simulink model "F16_aero"  (Simulink 7.2)
settings: Solver=ode45  StartTime=0.0  StopTime=10.0  RelTol=1e-3
model workspace (MAT data in the model file):
  F16_aero_data.ALPHA1_pts = [-10 -5 0 5 10 15 20 25 30 35 40 45]
  F16_aero_data.CX_table = [-0.099  -0.081  -0.081  -0.063  -0.025  0.044  0.097  0.113  0.145  0.167  0.174  0.166; -0.048  -0.038  -0.04  -0.021  0.016  0.083  0.127  0.137  0.162  0.177  0.179  0.167; -0.022  -0.02  -0.021  -0.004  0.032  0.094  0.128  0.13  0.154  0.161  0.155  0.138; -0.04  -0.038  -0.039  -0.025  0.006  0.062  0.087  0.085  0.1  0.11  0.104  0.091; -0.083  -0.073  -0.076  -0.072  -0.046  0.012  0.024  0.025  0.043  0.053  0.047  0.04]
  F16_aero_data.CZ0_table = [0.77 0.241 -0.1 -0.416 -0.731 -1.053 -1.366 -1.646 -1.917 -2.12 -2.248 -2.229]
  F16_aero_data.Cm0_table = [0.205  0.168  0.186  0.196  0.213  0.251  0.245  0.238  0.252  0.231  0.198  0.192; 0.081  0.077  0.107  0.11  0.11  0.141  0.127  0.119  0.133  0.108  0.081  0.093; -0.046  -0.02  -0.009  -0.005  -0.006  0.01  0.006  -0.001  0.014  0  -0.013  0.032; -0.174  -0.145  -0.121  -0.127  -0.129  -0.102  -0.097  -0.113  -0.087  -0.084  -0.069  -0.006; -0.259  -0.202  -0.184  -0.193  -0.199  -0.15  -0.16  -0.167  -0.104  -0.076  -0.041  -0.005]
  F16_aero_data.Cl0_table = [0  0  0  0  0  0  0  0  0  0  0  0; -0.001  -0.004  -0.008  -0.012  -0.016  -0.022  -0.022  -0.021  -0.015  -0.008  -0.013  -0.015; -0.003  -0.009  -0.017  -0.024  -0.03  -0.041  -0.045  -0.04  -0.016  -0.002  -0.01  -0.019; -0.001  -0.01  -0.02  -0.03  -0.039  -0.054  -0.057  -0.054  -0.023  -0.006  -0.014  -0.027; 0  -0.01  -0.022  -0.034  -0.047  -0.06  -0.069  -0.067  -0.033  -0.036  -0.035  -0.035; 0.007  -0.01  -0.023  -0.034  -0.049  -0.063  -0.081  -0.079  -0.06  -0.058  -0.062  -0.059; 0.009  -0.011  -0.023  -0.037  -0.05  -0.068  -0.089  -0.088  -0.091  -0.076  -0.077  -0.076]
  F16_aero_data.Cn0_table = [0  0  0  0  0  0  0  0  0  0  0  0; 0.018  0.019  0.018  0.019  0.019  0.018  0.013  0.007  0.004  -0.014  -0.017  -0.033; 0.038  0.042  0.042  0.042  0.043  0.039  0.03  0.017  0.004  -0.035  -0.047  -0.057; 0.056  0.057  0.059  0.058  0.058  0.053  0.032  0.012  0.002  -0.046  -0.071  -0.073; 0.064  0.077  0.076  0.074  0.073  0.057  0.029  0.007  0.012  -0.034  -0.065  -0.041; 0.074  0.086  0.093  0.089  0.08  0.062  0.049  0.022  0.028  -0.012  -0.002  -0.013; 0.079  0.09  0.106  0.106  0.096  0.08  0.068  0.03  0.064  0.015  0.011  -0.001]
  F16_aero_data.CXq_table = [-0.267 -0.11 0.308 1.34 2.08 2.91 2.76 2.05 1.5 1.49 1.83 1.21]
  F16_aero_data.CYr_table = [0.882 0.852 0.876 0.958 0.962 0.974 0.819 0.483 0.59 1.21 -0.493 -1.04]
  F16_aero_data.CYp_table = [-0.108 -0.108 -0.188 0.11 0.258 0.226 0.344 0.362 0.611 0.529 0.298 -0.227]
  F16_aero_data.CZq_table = [-8.8 -25.8 -28.9 -31.4 -31.2 -30.7 -27.7 -28.2 -29 -29.8 -38.3 -35.3]
  F16_aero_data.Clr_table = [-0.126 -0.026 0.063 0.113 0.208 0.23 0.319 0.437 0.68 0.1 0.447 -0.33]
  F16_aero_data.Clp_table = [-0.36 -0.359 -0.443 -0.42 -0.383 -0.375 -0.329 -0.294 -0.23 -0.21 -0.12 -0.1]
  F16_aero_data.Cmq_table = [-7.21 -5.4 -5.23 -5.26 -6.11 -6.64 -5.69 -6 -6.2 -6.4 -6.6 -6]
  F16_aero_data.Cnr_table = [-0.38 -0.363 -0.378 -0.386 -0.37 -0.453 -0.55 -0.582 -0.595 -0.637 -1.02 -0.84]
  F16_aero_data.Cnp_table = [0.061 0.052 0.052 -0.012 -0.013 -0.024 0.05 0.15 0.13 0.158 0.24 0.15]
  F16_aero_data.dlda_table = [-0.041  -0.052  -0.053  -0.056  -0.05  -0.056  -0.082  -0.059  -0.042  -0.038  -0.027  -0.017; -0.041  -0.053  -0.053  -0.053  -0.05  -0.051  -0.066  -0.043  -0.038  -0.027  -0.023  -0.016; -0.042  -0.053  -0.052  -0.051  -0.049  -0.049  -0.043  -0.035  -0.026  -0.016  -0.018  -0.014; -0.04  -0.052  -0.051  -0.052  -0.048  -0.048  -0.042  -0.037  -0.031  -0.026  -0.017  -0.012; -0.043  -0.049  -0.048  -0.049  -0.043  -0.042  -0.042  -0.036  -0.025  -0.021  -0.016  -0.011; -0.044  -0.048  -0.048  -0.047  -0.042  -0.041  -0.02  -0.028  -0.013  -0.014  -0.011  -0.01; -0.043  -0.049  -0.047  -0.045  -0.042  -0.037  -0.003  -0.013  -0.01  -0.003  -0.007  -0.008]
  F16_aero_data.dldr_table = [0.005  0.017  0.014  0.01  -0.005  0.009  0.019  0.005  0  -0.005  -0.011  0.008; 0.007  0.016  0.014  0.014  0.013  0.009  0.012  0.005  0  0.004  0.009  0.007; 0.013  0.013  0.011  0.012  0.011  0.009  0.008  0.005  0  0.005  0.003  0.005; 0.018  0.015  0.015  0.014  0.014  0.014  0.014  0.015  0.013  0.011  0.006  0.001; 0.015  0.014  0.013  0.013  0.012  0.011  0.011  0.01  0.008  0.008  0.007  0.003; 0.021  0.011  0.01  0.011  0.01  0.009  0.008  0.01  0.006  0.005  0  0.001; 0.023  0.01  0.011  0.011  0.011  0.01  0.008  0.01  0.006  0.014  0.02  0]
  F16_aero_data.dnda_table = [0.001  -0.027  -0.017  -0.013  -0.012  -0.016  0.001  0.017  0.011  0.017  0.008  0.016; 0.002  -0.014  -0.016  -0.016  -0.014  -0.019  -0.021  0.002  0.012  0.016  0.015  0.011; -0.006  -0.008  -0.006  -0.006  -0.005  -0.008  -0.005  0.007  0.004  0.007  0.006  0.006; -0.011  -0.011  -0.01  -0.009  -0.008  -0.006  0  0.004  0.007  0.01  0.004  0.01; -0.015  -0.015  -0.014  -0.012  -0.011  -0.008  -0.002  0.002  0.006  0.012  0.011  0.011; -0.024  -0.01  -0.004  -0.002  -0.001  0.003  0.014  0.006  -0.001  0.004  0.004  0.006; -0.022  0.002  -0.003  -0.005  -0.003  -0.001  -0.009  -0.009  -0.001  0.003  -0.002  0.001]
  F16_aero_data.dndr_table = [-0.018  -0.052  -0.052  -0.052  -0.054  -0.049  -0.059  -0.051  -0.03  -0.037  -0.026  -0.013; -0.028  -0.051  -0.043  -0.046  -0.045  -0.049  -0.057  -0.052  -0.03  -0.033  -0.03  -0.008; -0.037  -0.041  -0.038  -0.04  -0.04  -0.038  -0.037  -0.03  -0.027  -0.024  -0.019  -0.013; -0.048  -0.045  -0.045  -0.045  -0.044  -0.045  -0.047  -0.048  -0.049  -0.045  -0.033  -0.016; -0.043  -0.044  -0.041  -0.041  -0.04  -0.038  -0.034  -0.035  -0.035  -0.029  -0.022  -0.009; -0.052  -0.034  -0.036  -0.036  -0.035  -0.028  -0.024  -0.023  -0.02  -0.016  -0.01  -0.014; -0.062  -0.034  -0.027  -0.028  -0.027  -0.027  -0.023  -0.023  -0.019  -0.009  -0.025  -0.01]
  F16_aero_data.BETA2_pts = [-30 -20 -10 0 10 20 30]
  F16_aero_data.BETA1_pts = [0 5 10 15 20 25 30]
  F16_aero_data.DE1_pts : numeric (value not decoded)
libraries: simulink_need_slupdate x22
settings Model: Creator=bjax  LastModifiedBy=bjax

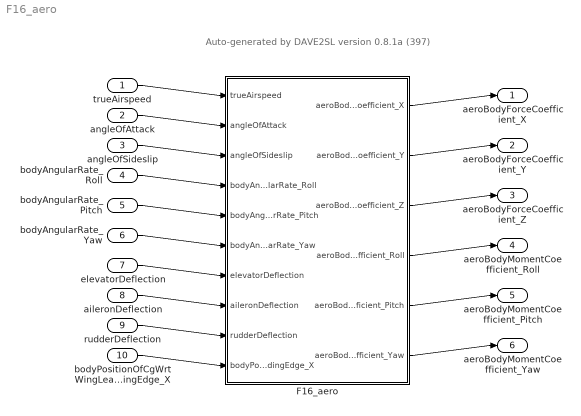
== system F16_aero ==
  note: Auto-generated by DAVE2SL version 0.8.1a (397)
  trueAirspeed : Inport
  angleOfAttack : Inport  Port=2
  angleOfSideslip : Inport  Port=3
  bodyAngularRate_Roll : Inport  Port=4
  bodyAngularRate_Pitch : Inport  Port=5
  bodyAngularRate_Yaw : Inport  Port=6
  elevatorDeflection : Inport  Port=7
  aileronDeflection : Inport  Port=8
  rudderDeflection : Inport  Port=9
  bodyPositionOfCgWrtWingLeadingEdge_X : Inport  Port=10
  F16_aero : Subsystem
  aeroBodyForceCoefficient_X : Outport
  aeroBodyForceCoefficient_Y : Outport  Port=2
  aeroBodyForceCoefficient_Z : Outport  Port=3
  aeroBodyMomentCoefficient_Roll : Outport  Port=4
  aeroBodyMomentCoefficient_Pitch : Outport  Port=5
  aeroBodyMomentCoefficient_Yaw : Outport  Port=6
  wires:
  trueAirspeed/1 -> F16_aero/1(trueAirspeed)
  angleOfAttack/1 -> F16_aero/2(angleOfAttack)
  angleOfSideslip/1 -> F16_aero/3(angleOfSideslip)
  bodyAngularRate_Roll/1 -> F16_aero/4(bodyAngularRate_Roll)
  bodyAngularRate_Pitch/1 -> F16_aero/5(bodyAngularRate_Pitch)
  bodyAngularRate_Yaw/1 -> F16_aero/6(bodyAngularRate_Yaw)
  elevatorDeflection/1 -> F16_aero/7(elevatorDeflection)
  aileronDeflection/1 -> F16_aero/8(aileronDeflection)
  rudderDeflection/1 -> F16_aero/9(rudderDeflection)
  bodyPositionOfCgWrtWingLeadingEdge_X/1 -> F16_aero/10(bodyPositionOfCgWrtWingLeadingEdge_X)
  F16_aero/1(aeroBodyForceCoefficient_X) -> aeroBodyForceCoefficient_X/1
  F16_aero/2(aeroBodyForceCoefficient_Y) -> aeroBodyForceCoefficient_Y/1
  F16_aero/3(aeroBodyForceCoefficient_Z) -> aeroBodyForceCoefficient_Z/1
  F16_aero/4(aeroBodyMomentCoefficient_Roll) -> aeroBodyMomentCoefficient_Roll/1
  F16_aero/5(aeroBodyMomentCoefficient_Pitch) -> aeroBodyMomentCoefficient_Pitch/1
  F16_aero/6(aeroBodyMomentCoefficient_Yaw) -> aeroBodyMomentCoefficient_Yaw/1

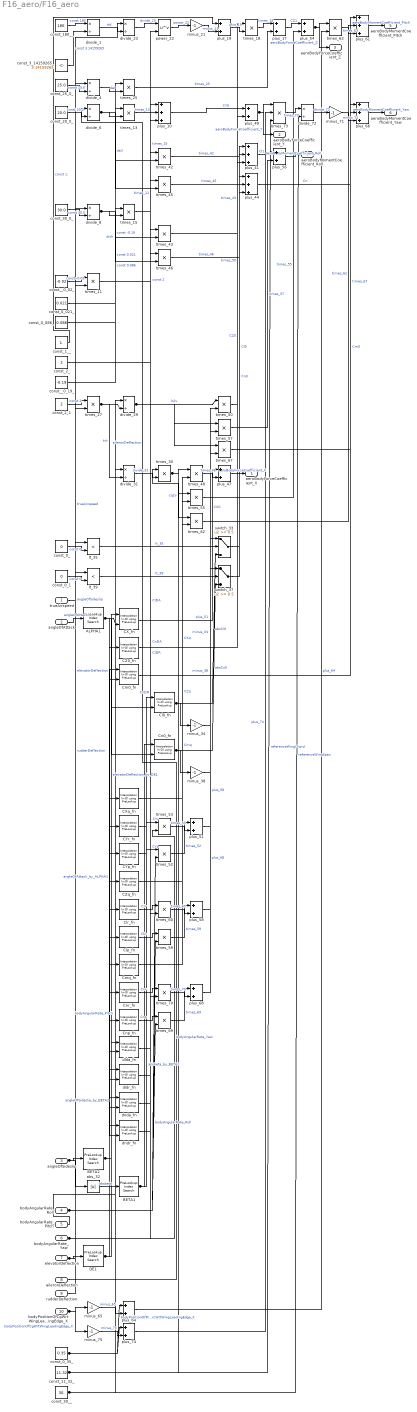
== system F16_aero/F16_aero ==
  trueAirspeed : Inport
  angleOfAttack : Inport  Port=2
  angleOfSideslip : Inport  Port=3
  bodyAngularRate_Roll : Inport  Port=4
  bodyAngularRate_Pitch : Inport  Port=5
  bodyAngularRate_Yaw : Inport  Port=6
  elevatorDeflection : Inport  Port=7
  aileronDeflection : Inport  Port=8
  rudderDeflection : Inport  Port=9
  bodyPositionOfCgWrtWingLeadingEdge_X : Inport  Port=10
  ALPHA1 : simulink_need_slupdate/PreLookup Index Search  bpData=F16_aero_data.ALPHA1_pts  searchMode=Binary Search  cacheBpFlag=on  outputFlag=off  IndexDataType=uint32  extrapMode=Linear Extrapolation  rangeErrorMode=None
  BETA1 : simulink_need_slupdate/PreLookup Index Search  bpData=F16_aero_data.BETA1_pts  searchMode=Binary Search  cacheBpFlag=on  outputFlag=off  IndexDataType=uint32  extrapMode=Linear Extrapolation  rangeErrorMode=None
  BETA2 : simulink_need_slupdate/PreLookup Index Search  bpData=F16_aero_data.BETA2_pts  searchMode=Binary Search  cacheBpFlag=on  outputFlag=off  IndexDataType=uint32  extrapMode=Linear Extrapolation  rangeErrorMode=None
  CX_fn : simulink_need_slupdate/Interpolation (n-D) using PreLookup  numDimsPopupSelect=2  explicitNumDims=2  table=F16_aero_data.CX_table  interpMethod=Linear  extrapMethod=None - Clip  rangeErrorMode=None  NumSelectionDims=0
  CXq_fn : simulink_need_slupdate/Interpolation (n-D) using PreLookup  numDimsPopupSelect=1  explicitNumDims=1  table=F16_aero_data.CXq_table  interpMethod=Linear  extrapMethod=None - Clip  rangeErrorMode=None  NumSelectionDims=0
  CYp_fn : simulink_need_slupdate/Interpolation (n-D) using PreLookup  numDimsPopupSelect=1  explicitNumDims=1  table=F16_aero_data.CYp_table  interpMethod=Linear  extrapMethod=None - Clip  rangeErrorMode=None  NumSelectionDims=0
  CYr_fn : simulink_need_slupdate/Interpolation (n-D) using PreLookup  numDimsPopupSelect=1  explicitNumDims=1  table=F16_aero_data.CYr_table  interpMethod=Linear  extrapMethod=None - Clip  rangeErrorMode=None  NumSelectionDims=0
  CZ0_fn : simulink_need_slupdate/Interpolation (n-D) using PreLookup  numDimsPopupSelect=1  explicitNumDims=1  table=F16_aero_data.CZ0_table  interpMethod=Linear  extrapMethod=None - Clip  rangeErrorMode=None  NumSelectionDims=0
  CZq_fn : simulink_need_slupdate/Interpolation (n-D) using PreLookup  numDimsPopupSelect=1  explicitNumDims=1  table=F16_aero_data.CZq_table  interpMethod=Linear  extrapMethod=None - Clip  rangeErrorMode=None  NumSelectionDims=0
  Cl0_fn : simulink_need_slupdate/Interpolation (n-D) using PreLookup  numDimsPopupSelect=2  explicitNumDims=2  table=F16_aero_data.Cl0_table  interpMethod=Linear  extrapMethod=None - Clip  rangeErrorMode=None  NumSelectionDims=0
  Clp_fn : simulink_need_slupdate/Interpolation (n-D) using PreLookup  numDimsPopupSelect=1  explicitNumDims=1  table=F16_aero_data.Clp_table  interpMethod=Linear  extrapMethod=None - Clip  rangeErrorMode=None  NumSelectionDims=0
  Clr_fn : simulink_need_slupdate/Interpolation (n-D) using PreLookup  numDimsPopupSelect=1  explicitNumDims=1  table=F16_aero_data.Clr_table  interpMethod=Linear  extrapMethod=None - Clip  rangeErrorMode=None  NumSelectionDims=0
  Cm0_fn : simulink_need_slupdate/Interpolation (n-D) using PreLookup  numDimsPopupSelect=2  explicitNumDims=2  table=F16_aero_data.Cm0_table  interpMethod=Linear  extrapMethod=None - Clip  rangeErrorMode=None  NumSelectionDims=0
  Cmq_fn : simulink_need_slupdate/Interpolation (n-D) using PreLookup  numDimsPopupSelect=1  explicitNumDims=1  table=F16_aero_data.Cmq_table  interpMethod=Linear  extrapMethod=None - Clip  rangeErrorMode=None  NumSelectionDims=0
  Cn0_fn : simulink_need_slupdate/Interpolation (n-D) using PreLookup  numDimsPopupSelect=2  explicitNumDims=2  table=F16_aero_data.Cn0_table  interpMethod=Linear  extrapMethod=None - Clip  rangeErrorMode=None  NumSelectionDims=0
  Cnp_fn : simulink_need_slupdate/Interpolation (n-D) using PreLookup  numDimsPopupSelect=1  explicitNumDims=1  table=F16_aero_data.Cnp_table  interpMethod=Linear  extrapMethod=None - Clip  rangeErrorMode=None  NumSelectionDims=0
  Cnr_fn : simulink_need_slupdate/Interpolation (n-D) using PreLookup  numDimsPopupSelect=1  explicitNumDims=1  table=F16_aero_data.Cnr_table  interpMethod=Linear  extrapMethod=None - Clip  rangeErrorMode=None  NumSelectionDims=0
  DE1 : simulink_need_slupdate/PreLookup Index Search  bpData=F16_aero_data.DE1_pts  searchMode=Binary Search  cacheBpFlag=on  outputFlag=off  IndexDataType=uint32  extrapMode=Linear Extrapolation  rangeErrorMode=None
  abs_32 : Abs  SaturateOnIntegerOverflow=on
  const_0_ : Constant  Value=0
  const_0_021_ : Constant  Value=0.021
  const_0_086_ : Constant  Value=0.086
  const_0_1 : Constant  Value=0
  const_0_35_ : Constant  Value=0.35
  const_11_32_ : Constant  Value=11.32
  const_180__ : Constant  Value=180.
  const_1__ : Constant  Value=1.
  const_20_0_ : Constant  Value=20.0
  const_25_0_ : Constant  Value=25.0
  const_2_ : Constant  Value=2
  const_2_1 : Constant  Value=2
  const_30_0_ : Constant  Value=30.0
  const_30__ : Constant  Value=30.
  const_3_14159265_ : Constant  Value=3.14159265
  const__0_02_ : Constant  Value=-0.02
  const__0_19_ : Constant  Value=-0.19
  divide_{1,4,6,8,23,29,31,72} (8 alike) : Product  Inputs=*/  SaturateOnIntegerOverflow=on  RndMeth=Zero  InputSameDT=on  OutDataTypeStr=Inherit: Same as first input
  dlda_fn : simulink_need_slupdate/Interpolation (n-D) using PreLookup  numDimsPopupSelect=2  explicitNumDims=2  table=F16_aero_data.dlda_table  interpMethod=Linear  extrapMethod=None - Clip  rangeErrorMode=None  NumSelectionDims=0
  dldr_fn : simulink_need_slupdate/Interpolation (n-D) using PreLookup  numDimsPopupSelect=2  explicitNumDims=2  table=F16_aero_data.dldr_table  interpMethod=Linear  extrapMethod=None - Clip  rangeErrorMode=None  NumSelectionDims=0
  dnda_fn : simulink_need_slupdate/Interpolation (n-D) using PreLookup  numDimsPopupSelect=2  explicitNumDims=2  table=F16_aero_data.dnda_table  interpMethod=Linear  extrapMethod=None - Clip  rangeErrorMode=None  NumSelectionDims=0
  dndr_fn : simulink_need_slupdate/Interpolation (n-D) using PreLookup  numDimsPopupSelect=2  explicitNumDims=2  table=F16_aero_data.dndr_table  interpMethod=Linear  extrapMethod=None - Clip  rangeErrorMode=None  NumSelectionDims=0
  lt_35 : RelationalOperator  Operator=<  InputSameDT=on
  lt_39 : RelationalOperator  Operator=<  InputSameDT=on
  minus_{21,34,38,65,71,75} (6 alike) : Gain  Gain=-1  SaturateOnIntegerOverflow=on  OutDataTypeStr=Inherit: Same as input  ParamDataTypeStr=Inherit: Same as input
  plus_{10,41,44,61,66} (5 alike) : Sum  Inputs=+++  SaturateOnIntegerOverflow=on  InputSameDT=on  OutDataTypeStr=Inherit: Same as first input
  plus_{17,19,47,49,51,54,56,58,64,68,74} (11 alike) : Sum  SaturateOnIntegerOverflow=on  InputSameDT=on  OutDataTypeStr=Inherit: Same as first input
  power_22 : Math  Operator=pow  SaturateOnIntegerOverflow=on
  switch_33 : Switch  Threshold=0.5  SaturateOnIntegerOverflow=on  InputSameDT=on
  switch_37 : Switch  Threshold=0.5  SaturateOnIntegerOverflow=on  InputSameDT=on
  times_{11,13,15,18,25,27,30,42..43,45..46,48,50,52..53,55,57,59..60,62..63,67,69..70} (24 alike) : Product  SaturateOnIntegerOverflow=on  RndMeth=Zero  InputSameDT=on  OutDataTypeStr=Inherit: Same as first input
  times_73 : Product  Inputs=3  SaturateOnIntegerOverflow=on  RndMeth=Zero  InputSameDT=on  OutDataTypeStr=Inherit: Same as first input
  aeroBodyForceCoefficient_X : Outport
  aeroBodyForceCoefficient_Y : Outport  Port=2
  aeroBodyForceCoefficient_Z : Outport  Port=3
  aeroBodyMomentCoefficient_Roll : Outport  Port=4
  aeroBodyMomentCoefficient_Pitch : Outport  Port=5
  aeroBodyMomentCoefficient_Yaw : Outport  Port=6
  wires:
  trueAirspeed/1 -> times_27/2  "trueAirspeed"
  angleOfAttack/1 -> ALPHA1/1  "angleOfAttack"
  angleOfSideslip/1 -> BETA2/1, times_11/2, divide_23/1, abs_32/1, lt_35/1, lt_39/1  "angleOfSideslip"
  bodyAngularRate_Roll/1 -> times_52/2, times_59/2, times_69/2  "bodyAngularRate_Roll"
  bodyAngularRate_Pitch/1 -> divide_31/1  "bodyAngularRate_Pitch"
  bodyAngularRate_Yaw/1 -> times_53/2, times_60/2, times_70/2  "bodyAngularRate_Yaw"
  elevatorDeflection/1 -> DE1/1, divide_4/1  "elevatorDeflection"
  aileronDeflection/1 -> divide_6/1  "aileronDeflection"
  rudderDeflection/1 -> divide_8/1  "rudderDeflection"
  bodyPositionOfCgWrtWingLeadingEdge_X/1 -> minus_65/1, minus_75/1  "bodyPositionOfCgWrtWingLeadingEdge_X"
  divide_1/1 -> divide_23/2  "rtd"
  const_180__/1 -> divide_1/1  "const 180."
  const_3_14159265_/1 -> divide_1/2  "const 3.14159265"
  const_0_35_/1 -> plus_64/1, plus_74/1  "bodyPositionOfMrcWrtWingLeadingEdge_X"
  const_11_32_/1 -> times_30/1, times_73/3  "referenceWingChord"
  const_30__/1 -> divide_29/1, divide_72/2  "referenceWingSpan"
  divide_4/1 -> times_25/2  "del"
  const_25_0_/1 -> divide_4/2  "const 25.0"
  divide_6/1 -> times_13/2, times_42/2, times_45/2  "dail"
  const_20_0_/1 -> divide_6/2  "const 20.0"
  divide_8/1 -> times_15/2, times_43/2, times_46/2  "drdr"
  const_30_0_/1 -> divide_8/2  "const 30.0"
  CX_fn/1 -> plus_47/1  "CX0"
  plus_10/1 -> plus_49/1  "CY0"
  times_11/1 -> plus_10/1  "times_11"
  const__0_02_/1 -> times_11/1  "const -0.02"
  times_13/1 -> plus_10/2  "times_13"
  const_0_021_/1 -> times_13/1  "const 0.021"
  times_15/1 -> plus_10/3  "times_15"
  const_0_086_/1 -> times_15/1  "const 0.086"
  CZ0_fn/1 -> times_18/1  "CZ0"
  plus_17/1 -> plus_54/1  "CZ1"
  times_18/1 -> plus_17/1  "times_18"
  plus_19/1 -> times_18/2  "plus_19"
  const_1__/1 -> plus_19/1  "const 1."
  minus_21/1 -> plus_19/2  "minus_21"
  power_22/1 -> minus_21/1  "power_22"
  divide_23/1 -> power_22/1  "divide_23"
  const_2_/1 -> power_22/2  "const 2"
  times_25/1 -> plus_17/2  "times_25"
  const__0_19_/1 -> times_25/1  "const -0.19"
  times_27/1 -> divide_29/2, divide_31/2  "tvt"
  const_2_1/1 -> times_27/1  "const 2"
  divide_29/1 -> times_50/1, times_57/1, times_67/1  "b2v"
  times_30/1 -> times_48/1, times_55/1, times_62/1  "cq2v"
  divide_31/1 -> times_30/2  "divide_31"
  abs_32/1 -> BETA1/1  "absbeta"
  Cl0_fn/1 -> switch_33/3, minus_34/1  "absCl0"
  Cn0_fn/1 -> switch_37/3, minus_38/1  "absCn0"
  switch_33/1 -> plus_41/1  "Cl0"
  minus_34/1 -> switch_33/1  "minus_34"
  lt_35/1 -> switch_33/2  "lt_35"
  const_0_/1 -> lt_35/2  "const 0"
  Cm0_fn/1 -> plus_61/1  "Cm0"
  switch_37/1 -> plus_44/1  "Cn0"
  minus_38/1 -> switch_37/1  "minus_38"
  lt_39/1 -> switch_37/2  "lt_39"
  const_0_1/1 -> lt_39/2  "const 0"
  CXq_fn/1 -> times_48/2  "CXq"
  CYr_fn/1 -> times_53/1  "CYr"
  CYp_fn/1 -> times_52/1  "CYp"
  CZq_fn/1 -> times_55/2  "CZq"
  Clr_fn/1 -> times_60/1  "Clr"
  Clp_fn/1 -> times_59/1  "Clp"
  Cmq_fn/1 -> times_62/2  "Cmq"
  Cnr_fn/1 -> times_70/1  "Cnr"
  Cnp_fn/1 -> times_69/1  "Cnp"
  dlda_fn/1 -> times_42/1  "ClDA"
  dldr_fn/1 -> times_43/1  "ClDR"
  dnda_fn/1 -> times_45/1  "CnDA"
  dndr_fn/1 -> times_46/1  "CnDR"
  plus_41/1 -> plus_56/1  "Cl1"
  times_42/1 -> plus_41/2  "times_42"
  times_43/1 -> plus_41/3  "times_43"
  plus_44/1 -> plus_66/1  "Cn"
  times_45/1 -> plus_44/2  "times_45"
  times_46/1 -> plus_44/3  "times_46"
  plus_47/1 -> aeroBodyForceCoefficient_X/1  "aeroBodyForceCoefficient_X"
  times_48/1 -> plus_47/2  "times_48"
  plus_49/1 -> times_73/1, aeroBodyForceCoefficient_Y/1  "aeroBodyForceCoefficient_Y"
  times_50/1 -> plus_49/2  "times_50"
  plus_51/1 -> times_50/2  "plus_51"
  times_52/1 -> plus_51/1  "times_52"
  times_53/1 -> plus_51/2  "times_53"
  plus_54/1 -> times_63/1, aeroBodyForceCoefficient_Z/1  "aeroBodyForceCoefficient_Z"
  times_55/1 -> plus_54/2  "times_55"
  plus_56/1 -> aeroBodyMomentCoefficient_Roll/1  "aeroBodyMomentCoefficient_Roll"
  times_57/1 -> plus_56/2  "times_57"
  plus_58/1 -> times_57/2  "plus_58"
  times_59/1 -> plus_58/1  "times_59"
  times_60/1 -> plus_58/2  "times_60"
  plus_61/1 -> aeroBodyMomentCoefficient_Pitch/1  "aeroBodyMomentCoefficient_Pitch"
  times_62/1 -> plus_61/2  "times_62"
  times_63/1 -> plus_61/3  "times_63"
  plus_64/1 -> times_63/2  "plus_64"
  minus_65/1 -> plus_64/2  "minus_65"
  plus_66/1 -> aeroBodyMomentCoefficient_Yaw/1  "aeroBodyMomentCoefficient_Yaw"
  times_67/1 -> plus_66/2  "times_67"
  plus_68/1 -> times_67/2  "plus_68"
  times_69/1 -> plus_68/1  "times_69"
  times_70/1 -> plus_68/2  "times_70"
  minus_71/1 -> plus_66/3  "minus_71"
  divide_72/1 -> minus_71/1  "divide_72"
  times_73/1 -> divide_72/1  "times_73"
  plus_74/1 -> times_73/2  "plus_74"
  minus_75/1 -> plus_74/2  "minus_75"
  DE1/1 -> CX_fn/1, Cm0_fn/1  "elevatorDeflection_by_DE1"
  ALPHA1/1 -> CX_fn/2, CZ0_fn/1, Cm0_fn/2, Cl0_fn/2, Cn0_fn/2, CXq_fn/1, CYr_fn/1, CYp_fn/1, CZq_fn/1, Clr_fn/1, Clp_fn/1, Cmq_fn/1, Cnr_fn/1, Cnp_fn/1, dlda_fn/2, dldr_fn/2, dnda_fn/2, dndr_fn/2  "angleOfAttack_by_ALPHA1"
  BETA1/1 -> Cl0_fn/1, Cn0_fn/1  "absbeta_by_BETA1"
  BETA2/1 -> dlda_fn/1, dldr_fn/1, dnda_fn/1, dndr_fn/1  "angleOfSideslip_by_BETA2"
